simulink model "SimpleBattery"  (R2021a)
settings: Solver=VariableStepAuto  StartTime=0.0  StopTime=sim_time  RelTol=1e-3
values from neighbouring files (symbols this model uses):
  Cn = 5.4 * 3600    (= 19440)    [CombinedBattery.m]    (also in OCV_PRC.m; SimpleBatteryDischarging_run.m = 8280; SimpleBattery_run.m = 8280)
  I = -1 * I    [CombinedBattery.m]    (also in OCV_PRC.m = -1*I; SimpleBatteryDischarging_run.m = 2.3; SimpleBattery_run.m = -2.3)
  OCV = 3    [CombinedBattery.m]    (also in SimpleBatteryDischarging_run.m = Battery_Data(:,2); SimpleBattery_run.m = Battery_Data(:,2))
  R_Charging = Battery_Data(:,3)    [SimpleBatteryDischarging_run.m]    (also in SimpleBattery_run.m)
  R_Discharging = Battery_Data(:,4)    [SimpleBatteryDischarging_run.m]    (also in SimpleBattery_run.m)
  SOC = SOC - (DeltaT * I(k) / Cn)    [CombinedBattery.m]    (also in OCV_PRC.m = SOC - (DeltaT/Cn) * I(k); SimpleBatteryDischarging_run.m = Battery_Data(:,1); SimpleBattery_run.m = Battery_Data(:,1))
settings Model: Creator=shinyh  LastModifiedBy=shinyh

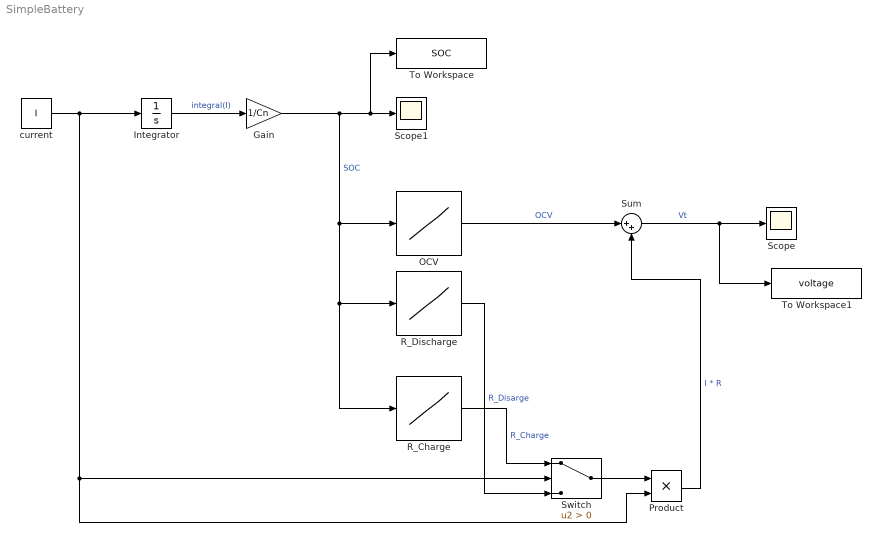
== system SimpleBattery ==
  Gain : Gain  Gain=1/Cn
  Integrator : Integrator
  OCV : Lookup_n-D  NumberOfTableDimensions=1  BreakpointsForDimension1=SOC  Table=OCV  InternalRulePriority=Speed  RndMeth=Simplest  InputSameDT=on
  Product : Product
  R_Charge : Lookup_n-D  NumberOfTableDimensions=1  BreakpointsForDimension1=SOC  Table=R_Charging  InternalRulePriority=Speed  RndMeth=Simplest  InputSameDT=on
  R_Discharge : Lookup_n-D  NumberOfTableDimensions=1  BreakpointsForDimension1=SOC  Table=R_Discharging  InternalRulePriority=Speed  RndMeth=Simplest  InputSameDT=on
  Scope : Scope
  Scope1 : Scope
  Sum : Sum  Inputs=|++
  Switch : Switch  Criteria=u2 > Threshold
  To Workspace : ToWorkspace  VariableName=SOC  SaveFormat=Timeseries  SampleTime=-1
  To Workspace1 : ToWorkspace  VariableName=voltage  SaveFormat=Timeseries  SampleTime=-1
  current : Constant  Value=I
  wires:
  current/1 -> Product/2, Switch/2, Integrator/1
  Integrator/1 -> Gain/1  "integral(I)"
  Gain/1 -> To Workspace/1, Scope1/1, R_Charge/1, R_Discharge/1, OCV/1  "SOC"
  OCV/1 -> Sum/1  "OCV"
  Product/1 -> Sum/2  "I * R"
  Sum/1 -> To Workspace1/1, Scope/1  "Vt"
  Switch/1 -> Product/1
  R_Charge/1 -> Switch/1  "R_Charge"
  R_Discharge/1 -> Switch/3  "R_Disarge"
